simulink model "workingGT3nomasknwithcontrol"  (R2024a)
settings: Solver=ode15s  StartTime=0.0  StopTime=3600*48  RelTol=0.0001
model workspace (MAT data in the model file):
  TempGrad = 15
  Ti = 5
  roomarea1 = 20
libraries: fl_lib x2433, nesl_utility x241, SimscapeFluids_lib x137
(part 41 of 41)

== system workingGT3nomasknwithcontrol/OG2/Raum11/Heater/Controller fbh ==
  Temp : Inport
  Constant2 : Constant  Value=-1
  Product2 : Product
  Relay1 : Relay  OnSwitchValue=-19  OffSwitchValue=-21  OnOutputValue=.098  OffOutputValue=0.00001
  Simulink-PS Converter1 : nesl_utility/Simulink-PS Converter  PhysicalDomain=network_engine_domain  SubClassName=ps_input  LeftPortType=input  RightPortType=output  PseudoPeriodic=off  Frequencies=[]  NoiseDistribution=none  NoiseParameters=[]  Unit=1  AffineConversion=off  FilteringAndDerivatives=provide  SimscapeFilterOrder=1  InputFilterTimeConstant=0.001  UdotUserProvided=0
  output : PMIOPort  Side=Right
  wires:
  Constant2/1 -> Product2/2
  Temp/1 -> Product2/1
  Product2/1 -> Relay1/1
  Relay1/1 -> Simulink-PS Converter1/1
  connections:
  Simulink-PS Converter1/RConn1 -- output/RConn1

== system workingGT3nomasknwithcontrol/OG2/Raum12/Heater/Controller 11 ==
  In1 : Inport
  Constant2 : Constant  Value=-1
  Product2 : Product
  Relay1 : Relay  OnSwitchValue=-19  OffSwitchValue=-21  OnOutputValue=.095  OffOutputValue=0.00001
  Simulink-PS Converter1 : nesl_utility/Simulink-PS Converter  PhysicalDomain=network_engine_domain  SubClassName=ps_input  LeftPortType=input  RightPortType=output  PseudoPeriodic=off  Frequencies=[]  NoiseDistribution=none  NoiseParameters=[]  Unit=1  AffineConversion=off  FilteringAndDerivatives=provide  SimscapeFilterOrder=1  InputFilterTimeConstant=0.001  UdotUserProvided=0
  output : PMIOPort  Side=Right
  wires:
  Constant2/1 -> Product2/2
  In1/1 -> Product2/1
  Product2/1 -> Relay1/1
  Relay1/1 -> Simulink-PS Converter1/1
  connections:
  Simulink-PS Converter1/RConn1 -- output/RConn1

== system workingGT3nomasknwithcontrol/OG2/Raum12/Heater/Controller 22 ==
  Temp : Inport
  Constant2 : Constant  Value=-1
  Product2 : Product
  Relay1 : Relay  OnSwitchValue=-19  OffSwitchValue=-21  OnOutputValue=.098  OffOutputValue=0.00001
  Simulink-PS Converter1 : nesl_utility/Simulink-PS Converter  PhysicalDomain=network_engine_domain  SubClassName=ps_input  LeftPortType=input  RightPortType=output  PseudoPeriodic=off  Frequencies=[]  NoiseDistribution=none  NoiseParameters=[]  Unit=1  AffineConversion=off  FilteringAndDerivatives=provide  SimscapeFilterOrder=1  InputFilterTimeConstant=0.001  UdotUserProvided=0
  output : PMIOPort  Side=Right
  wires:
  Relay1/1 -> Simulink-PS Converter1/1
  Product2/1 -> Relay1/1
  Temp/1 -> Product2/1
  Constant2/1 -> Product2/2
  connections:
  Simulink-PS Converter1/RConn1 -- output/RConn1

== system workingGT3nomasknwithcontrol/OG2/Raum12/Heater/Controller 33 ==
  Temp : Inport
  Constant2 : Constant  Value=-1
  Product2 : Product
  Relay1 : Relay  OnSwitchValue=-19  OffSwitchValue=-21  OnOutputValue=.098  OffOutputValue=0.00001
  Simulink-PS Converter1 : nesl_utility/Simulink-PS Converter  PhysicalDomain=network_engine_domain  SubClassName=ps_input  LeftPortType=input  RightPortType=output  PseudoPeriodic=off  Frequencies=[]  NoiseDistribution=none  NoiseParameters=[]  Unit=1  AffineConversion=off  FilteringAndDerivatives=provide  SimscapeFilterOrder=1  InputFilterTimeConstant=0.001  UdotUserProvided=0
  output : PMIOPort  Side=Right
  wires:
  Constant2/1 -> Product2/2
  Temp/1 -> Product2/1
  Product2/1 -> Relay1/1
  Relay1/1 -> Simulink-PS Converter1/1
  connections:
  Simulink-PS Converter1/RConn1 -- output/RConn1

== system workingGT3nomasknwithcontrol/OG2/Raum12/Heater/Controller fbh ==
  Temp : Inport
  Constant2 : Constant  Value=-1
  Product2 : Product
  Relay1 : Relay  OnSwitchValue=-19  OffSwitchValue=-21  OnOutputValue=.098  OffOutputValue=0.00001
  Simulink-PS Converter1 : nesl_utility/Simulink-PS Converter  PhysicalDomain=network_engine_domain  SubClassName=ps_input  LeftPortType=input  RightPortType=output  PseudoPeriodic=off  Frequencies=[]  NoiseDistribution=none  NoiseParameters=[]  Unit=1  AffineConversion=off  FilteringAndDerivatives=provide  SimscapeFilterOrder=1  InputFilterTimeConstant=0.001  UdotUserProvided=0
  output : PMIOPort  Side=Right
  wires:
  Relay1/1 -> Simulink-PS Converter1/1
  Product2/1 -> Relay1/1
  Temp/1 -> Product2/1
  Constant2/1 -> Product2/2
  connections:
  Simulink-PS Converter1/RConn1 -- output/RConn1

== system workingGT3nomasknwithcontrol/OG2/Raum2/Heater/Controller 11 ==
  In1 : Inport
  Constant2 : Constant  Value=-1
  Product2 : Product
  Relay1 : Relay  OnSwitchValue=-14  OffSwitchValue=-16  OnOutputValue=.095  OffOutputValue=0.00001
  Simulink-PS Converter1 : nesl_utility/Simulink-PS Converter  PhysicalDomain=network_engine_domain  SubClassName=ps_input  LeftPortType=input  RightPortType=output  PseudoPeriodic=off  Frequencies=[]  NoiseDistribution=none  NoiseParameters=[]  Unit=1  AffineConversion=off  FilteringAndDerivatives=provide  SimscapeFilterOrder=1  InputFilterTimeConstant=0.001  UdotUserProvided=0
  output : PMIOPort  Side=Right
  wires:
  Constant2/1 -> Product2/2
  In1/1 -> Product2/1
  Product2/1 -> Relay1/1
  Relay1/1 -> Simulink-PS Converter1/1
  connections:
  Simulink-PS Converter1/RConn1 -- output/RConn1

== system workingGT3nomasknwithcontrol/OG2/Raum2/Heater/Controller 22 ==
  Temp : Inport
  Constant2 : Constant  Value=-1
  Product2 : Product
  Relay1 : Relay  OnSwitchValue=-19  OffSwitchValue=-21  OnOutputValue=.098  OffOutputValue=0.00001
  Simulink-PS Converter1 : nesl_utility/Simulink-PS Converter  PhysicalDomain=network_engine_domain  SubClassName=ps_input  LeftPortType=input  RightPortType=output  PseudoPeriodic=off  Frequencies=[]  NoiseDistribution=none  NoiseParameters=[]  Unit=1  AffineConversion=off  FilteringAndDerivatives=provide  SimscapeFilterOrder=1  InputFilterTimeConstant=0.001  UdotUserProvided=0
  output : PMIOPort  Side=Right
  wires:
  Relay1/1 -> Simulink-PS Converter1/1
  Product2/1 -> Relay1/1
  Temp/1 -> Product2/1
  Constant2/1 -> Product2/2
  connections:
  Simulink-PS Converter1/RConn1 -- output/RConn1

== system workingGT3nomasknwithcontrol/OG2/Raum2/Heater/Controller 33 ==
  Temp : Inport
  Constant2 : Constant  Value=-1
  Product2 : Product
  Relay1 : Relay  OnSwitchValue=-19  OffSwitchValue=-21  OnOutputValue=.098  OffOutputValue=0.00001
  Simulink-PS Converter1 : nesl_utility/Simulink-PS Converter  PhysicalDomain=network_engine_domain  SubClassName=ps_input  LeftPortType=input  RightPortType=output  PseudoPeriodic=off  Frequencies=[]  NoiseDistribution=none  NoiseParameters=[]  Unit=1  AffineConversion=off  FilteringAndDerivatives=provide  SimscapeFilterOrder=1  InputFilterTimeConstant=0.001  UdotUserProvided=0
  output : PMIOPort  Side=Right
  wires:
  Constant2/1 -> Product2/2
  Temp/1 -> Product2/1
  Product2/1 -> Relay1/1
  Relay1/1 -> Simulink-PS Converter1/1
  connections:
  Simulink-PS Converter1/RConn1 -- output/RConn1

== system workingGT3nomasknwithcontrol/OG2/Raum2/Heater/Controller fbh ==
  Temp : Inport
  Constant2 : Constant  Value=-1
  Product2 : Product
  Relay1 : Relay  OnSwitchValue=-19  OffSwitchValue=-21  OnOutputValue=.098  OffOutputValue=0.00001
  Simulink-PS Converter1 : nesl_utility/Simulink-PS Converter  PhysicalDomain=network_engine_domain  SubClassName=ps_input  LeftPortType=input  RightPortType=output  PseudoPeriodic=off  Frequencies=[]  NoiseDistribution=none  NoiseParameters=[]  Unit=1  AffineConversion=off  FilteringAndDerivatives=provide  SimscapeFilterOrder=1  InputFilterTimeConstant=0.001  UdotUserProvided=0
  output : PMIOPort  Side=Right
  wires:
  Relay1/1 -> Simulink-PS Converter1/1
  Product2/1 -> Relay1/1
  Temp/1 -> Product2/1
  Constant2/1 -> Product2/2
  connections:
  Simulink-PS Converter1/RConn1 -- output/RConn1

== system workingGT3nomasknwithcontrol/OG2/Raum3/Heater/Controller 11 ==
  In1 : Inport
  Constant2 : Constant  Value=-1
  Product2 : Product
  Relay1 : Relay  OnSwitchValue=-19  OffSwitchValue=-21  OnOutputValue=.095  OffOutputValue=0.00001
  Simulink-PS Converter1 : nesl_utility/Simulink-PS Converter  PhysicalDomain=network_engine_domain  SubClassName=ps_input  LeftPortType=input  RightPortType=output  PseudoPeriodic=off  Frequencies=[]  NoiseDistribution=none  NoiseParameters=[]  Unit=1  AffineConversion=off  FilteringAndDerivatives=provide  SimscapeFilterOrder=1  InputFilterTimeConstant=0.001  UdotUserProvided=0
  output : PMIOPort  Side=Right
  wires:
  Relay1/1 -> Simulink-PS Converter1/1
  Product2/1 -> Relay1/1
  In1/1 -> Product2/1
  Constant2/1 -> Product2/2
  connections:
  Simulink-PS Converter1/RConn1 -- output/RConn1

== system workingGT3nomasknwithcontrol/OG2/Raum3/Heater/Controller 22 ==
  Temp : Inport
  Constant2 : Constant  Value=-1
  Product2 : Product
  Relay1 : Relay  OnSwitchValue=-19  OffSwitchValue=-21  OnOutputValue=.098  OffOutputValue=0.00001
  Simulink-PS Converter1 : nesl_utility/Simulink-PS Converter  PhysicalDomain=network_engine_domain  SubClassName=ps_input  LeftPortType=input  RightPortType=output  PseudoPeriodic=off  Frequencies=[]  NoiseDistribution=none  NoiseParameters=[]  Unit=1  AffineConversion=off  FilteringAndDerivatives=provide  SimscapeFilterOrder=1  InputFilterTimeConstant=0.001  UdotUserProvided=0
  output : PMIOPort  Side=Right
  wires:
  Constant2/1 -> Product2/2
  Temp/1 -> Product2/1
  Product2/1 -> Relay1/1
  Relay1/1 -> Simulink-PS Converter1/1
  connections:
  Simulink-PS Converter1/RConn1 -- output/RConn1

== system workingGT3nomasknwithcontrol/OG2/Raum3/Heater/Controller 33 ==
  Temp : Inport
  Constant2 : Constant  Value=-1
  Product2 : Product
  Relay1 : Relay  OnSwitchValue=-19  OffSwitchValue=-21  OnOutputValue=.098  OffOutputValue=0.00001
  Simulink-PS Converter1 : nesl_utility/Simulink-PS Converter  PhysicalDomain=network_engine_domain  SubClassName=ps_input  LeftPortType=input  RightPortType=output  PseudoPeriodic=off  Frequencies=[]  NoiseDistribution=none  NoiseParameters=[]  Unit=1  AffineConversion=off  FilteringAndDerivatives=provide  SimscapeFilterOrder=1  InputFilterTimeConstant=0.001  UdotUserProvided=0
  output : PMIOPort  Side=Right
  wires:
  Relay1/1 -> Simulink-PS Converter1/1
  Product2/1 -> Relay1/1
  Temp/1 -> Product2/1
  Constant2/1 -> Product2/2
  connections:
  Simulink-PS Converter1/RConn1 -- output/RConn1

== system workingGT3nomasknwithcontrol/OG2/Raum3/Heater/Controller fbh ==
  Temp : Inport
  Constant2 : Constant  Value=-1
  Product2 : Product
  Relay1 : Relay  OnSwitchValue=-19  OffSwitchValue=-21  OnOutputValue=.098  OffOutputValue=0.00001
  Simulink-PS Converter1 : nesl_utility/Simulink-PS Converter  PhysicalDomain=network_engine_domain  SubClassName=ps_input  LeftPortType=input  RightPortType=output  PseudoPeriodic=off  Frequencies=[]  NoiseDistribution=none  NoiseParameters=[]  Unit=1  AffineConversion=off  FilteringAndDerivatives=provide  SimscapeFilterOrder=1  InputFilterTimeConstant=0.001  UdotUserProvided=0
  output : PMIOPort  Side=Right
  wires:
  Constant2/1 -> Product2/2
  Temp/1 -> Product2/1
  Product2/1 -> Relay1/1
  Relay1/1 -> Simulink-PS Converter1/1
  connections:
  Simulink-PS Converter1/RConn1 -- output/RConn1

== system workingGT3nomasknwithcontrol/OG2/Raum4/Heater/Controller 11 ==
  In1 : Inport
  Constant2 : Constant  Value=-1
  Product2 : Product
  Relay1 : Relay  OnSwitchValue=-23  OffSwitchValue=-25  OnOutputValue=.095  OffOutputValue=0.00001
  Simulink-PS Converter1 : nesl_utility/Simulink-PS Converter  PhysicalDomain=network_engine_domain  SubClassName=ps_input  LeftPortType=input  RightPortType=output  PseudoPeriodic=off  Frequencies=[]  NoiseDistribution=none  NoiseParameters=[]  Unit=1  AffineConversion=off  FilteringAndDerivatives=provide  SimscapeFilterOrder=1  InputFilterTimeConstant=0.001  UdotUserProvided=0
  output : PMIOPort  Side=Right
  wires:
  Relay1/1 -> Simulink-PS Converter1/1
  Product2/1 -> Relay1/1
  In1/1 -> Product2/1
  Constant2/1 -> Product2/2
  connections:
  Simulink-PS Converter1/RConn1 -- output/RConn1

== system workingGT3nomasknwithcontrol/OG2/Raum4/Heater/Controller 22 ==
  Temp : Inport
  Constant2 : Constant  Value=-1
  Product2 : Product
  Relay1 : Relay  OnSwitchValue=-19  OffSwitchValue=-21  OnOutputValue=.098  OffOutputValue=0.00001
  Simulink-PS Converter1 : nesl_utility/Simulink-PS Converter  PhysicalDomain=network_engine_domain  SubClassName=ps_input  LeftPortType=input  RightPortType=output  PseudoPeriodic=off  Frequencies=[]  NoiseDistribution=none  NoiseParameters=[]  Unit=1  AffineConversion=off  FilteringAndDerivatives=provide  SimscapeFilterOrder=1  InputFilterTimeConstant=0.001  UdotUserProvided=0
  output : PMIOPort  Side=Right
  wires:
  Constant2/1 -> Product2/2
  Temp/1 -> Product2/1
  Product2/1 -> Relay1/1
  Relay1/1 -> Simulink-PS Converter1/1
  connections:
  Simulink-PS Converter1/RConn1 -- output/RConn1

== system workingGT3nomasknwithcontrol/OG2/Raum4/Heater/Controller 33 ==
  Temp : Inport
  Constant2 : Constant  Value=-1
  Product2 : Product
  Relay1 : Relay  OnSwitchValue=-19  OffSwitchValue=-21  OnOutputValue=.098  OffOutputValue=0.00001
  Simulink-PS Converter1 : nesl_utility/Simulink-PS Converter  PhysicalDomain=network_engine_domain  SubClassName=ps_input  LeftPortType=input  RightPortType=output  PseudoPeriodic=off  Frequencies=[]  NoiseDistribution=none  NoiseParameters=[]  Unit=1  AffineConversion=off  FilteringAndDerivatives=provide  SimscapeFilterOrder=1  InputFilterTimeConstant=0.001  UdotUserProvided=0
  output : PMIOPort  Side=Right
  wires:
  Relay1/1 -> Simulink-PS Converter1/1
  Product2/1 -> Relay1/1
  Temp/1 -> Product2/1
  Constant2/1 -> Product2/2
  connections:
  Simulink-PS Converter1/RConn1 -- output/RConn1

== system workingGT3nomasknwithcontrol/OG2/Raum4/Heater/Controller fbh ==
  Temp : Inport
  Constant2 : Constant  Value=-1
  Product2 : Product
  Relay1 : Relay  OnSwitchValue=-19  OffSwitchValue=-21  OnOutputValue=.098  OffOutputValue=0.00001
  Simulink-PS Converter1 : nesl_utility/Simulink-PS Converter  PhysicalDomain=network_engine_domain  SubClassName=ps_input  LeftPortType=input  RightPortType=output  PseudoPeriodic=off  Frequencies=[]  NoiseDistribution=none  NoiseParameters=[]  Unit=1  AffineConversion=off  FilteringAndDerivatives=provide  SimscapeFilterOrder=1  InputFilterTimeConstant=0.001  UdotUserProvided=0
  output : PMIOPort  Side=Right
  wires:
  Constant2/1 -> Product2/2
  Temp/1 -> Product2/1
  Product2/1 -> Relay1/1
  Relay1/1 -> Simulink-PS Converter1/1
  connections:
  Simulink-PS Converter1/RConn1 -- output/RConn1

== system workingGT3nomasknwithcontrol/OG2/Raum5/Heater/Controller 11 ==
  In1 : Inport
  Constant2 : Constant  Value=-1
  Product2 : Product
  Relay1 : Relay  OnSwitchValue=-19  OffSwitchValue=-21  OnOutputValue=.095  OffOutputValue=0.00001
  Simulink-PS Converter1 : nesl_utility/Simulink-PS Converter  PhysicalDomain=network_engine_domain  SubClassName=ps_input  LeftPortType=input  RightPortType=output  PseudoPeriodic=off  Frequencies=[]  NoiseDistribution=none  NoiseParameters=[]  Unit=1  AffineConversion=off  FilteringAndDerivatives=provide  SimscapeFilterOrder=1  InputFilterTimeConstant=0.001  UdotUserProvided=0
  output : PMIOPort  Side=Right
  wires:
  Constant2/1 -> Product2/2
  In1/1 -> Product2/1
  Product2/1 -> Relay1/1
  Relay1/1 -> Simulink-PS Converter1/1
  connections:
  Simulink-PS Converter1/RConn1 -- output/RConn1

== system workingGT3nomasknwithcontrol/OG2/Raum5/Heater/Controller 22 ==
  Temp : Inport
  Constant2 : Constant  Value=-1
  Product2 : Product
  Relay1 : Relay  OnSwitchValue=-19  OffSwitchValue=-21  OnOutputValue=.098  OffOutputValue=0.00001
  Simulink-PS Converter1 : nesl_utility/Simulink-PS Converter  PhysicalDomain=network_engine_domain  SubClassName=ps_input  LeftPortType=input  RightPortType=output  PseudoPeriodic=off  Frequencies=[]  NoiseDistribution=none  NoiseParameters=[]  Unit=1  AffineConversion=off  FilteringAndDerivatives=provide  SimscapeFilterOrder=1  InputFilterTimeConstant=0.001  UdotUserProvided=0
  output : PMIOPort  Side=Right
  wires:
  Relay1/1 -> Simulink-PS Converter1/1
  Product2/1 -> Relay1/1
  Temp/1 -> Product2/1
  Constant2/1 -> Product2/2
  connections:
  Simulink-PS Converter1/RConn1 -- output/RConn1

== system workingGT3nomasknwithcontrol/OG2/Raum5/Heater/Controller 33 ==
  Temp : Inport
  Constant2 : Constant  Value=-1
  Product2 : Product
  Relay1 : Relay  OnSwitchValue=-19  OffSwitchValue=-21  OnOutputValue=.098  OffOutputValue=0.00001
  Simulink-PS Converter1 : nesl_utility/Simulink-PS Converter  PhysicalDomain=network_engine_domain  SubClassName=ps_input  LeftPortType=input  RightPortType=output  PseudoPeriodic=off  Frequencies=[]  NoiseDistribution=none  NoiseParameters=[]  Unit=1  AffineConversion=off  FilteringAndDerivatives=provide  SimscapeFilterOrder=1  InputFilterTimeConstant=0.001  UdotUserProvided=0
  output : PMIOPort  Side=Right
  wires:
  Constant2/1 -> Product2/2
  Temp/1 -> Product2/1
  Product2/1 -> Relay1/1
  Relay1/1 -> Simulink-PS Converter1/1
  connections:
  Simulink-PS Converter1/RConn1 -- output/RConn1

== system workingGT3nomasknwithcontrol/OG2/Raum5/Heater/Controller fbh ==
  Temp : Inport
  Constant2 : Constant  Value=-1
  Product2 : Product
  Relay1 : Relay  OnSwitchValue=-19  OffSwitchValue=-21  OnOutputValue=.098  OffOutputValue=0.00001
  Simulink-PS Converter1 : nesl_utility/Simulink-PS Converter  PhysicalDomain=network_engine_domain  SubClassName=ps_input  LeftPortType=input  RightPortType=output  PseudoPeriodic=off  Frequencies=[]  NoiseDistribution=none  NoiseParameters=[]  Unit=1  AffineConversion=off  FilteringAndDerivatives=provide  SimscapeFilterOrder=1  InputFilterTimeConstant=0.001  UdotUserProvided=0
  output : PMIOPort  Side=Right
  wires:
  Relay1/1 -> Simulink-PS Converter1/1
  Product2/1 -> Relay1/1
  Temp/1 -> Product2/1
  Constant2/1 -> Product2/2
  connections:
  Simulink-PS Converter1/RConn1 -- output/RConn1

== system workingGT3nomasknwithcontrol/OG2/Raum6/Heater/Controller 11 ==
  In1 : Inport
  Constant2 : Constant  Value=-1
  Product2 : Product
  Relay1 : Relay  OnSwitchValue=-19  OffSwitchValue=-21  OnOutputValue=.095  OffOutputValue=0.00001
  Simulink-PS Converter1 : nesl_utility/Simulink-PS Converter  PhysicalDomain=network_engine_domain  SubClassName=ps_input  LeftPortType=input  RightPortType=output  PseudoPeriodic=off  Frequencies=[]  NoiseDistribution=none  NoiseParameters=[]  Unit=1  AffineConversion=off  FilteringAndDerivatives=provide  SimscapeFilterOrder=1  InputFilterTimeConstant=0.001  UdotUserProvided=0
  output : PMIOPort  Side=Right
  wires:
  Relay1/1 -> Simulink-PS Converter1/1
  Product2/1 -> Relay1/1
  In1/1 -> Product2/1
  Constant2/1 -> Product2/2
  connections:
  Simulink-PS Converter1/RConn1 -- output/RConn1

== system workingGT3nomasknwithcontrol/OG2/Raum6/Heater/Controller 22 ==
  Temp : Inport
  Constant2 : Constant  Value=-1
  Product2 : Product
  Relay1 : Relay  OnSwitchValue=-19  OffSwitchValue=-21  OnOutputValue=.098  OffOutputValue=0.00001
  Simulink-PS Converter1 : nesl_utility/Simulink-PS Converter  PhysicalDomain=network_engine_domain  SubClassName=ps_input  LeftPortType=input  RightPortType=output  PseudoPeriodic=off  Frequencies=[]  NoiseDistribution=none  NoiseParameters=[]  Unit=1  AffineConversion=off  FilteringAndDerivatives=provide  SimscapeFilterOrder=1  InputFilterTimeConstant=0.001  UdotUserProvided=0
  output : PMIOPort  Side=Right
  wires:
  Constant2/1 -> Product2/2
  Temp/1 -> Product2/1
  Product2/1 -> Relay1/1
  Relay1/1 -> Simulink-PS Converter1/1
  connections:
  Simulink-PS Converter1/RConn1 -- output/RConn1

== system workingGT3nomasknwithcontrol/OG2/Raum6/Heater/Controller 33 ==
  Temp : Inport
  Constant2 : Constant  Value=-1
  Product2 : Product
  Relay1 : Relay  OnSwitchValue=-19  OffSwitchValue=-21  OnOutputValue=.098  OffOutputValue=0.00001
  Simulink-PS Converter1 : nesl_utility/Simulink-PS Converter  PhysicalDomain=network_engine_domain  SubClassName=ps_input  LeftPortType=input  RightPortType=output  PseudoPeriodic=off  Frequencies=[]  NoiseDistribution=none  NoiseParameters=[]  Unit=1  AffineConversion=off  FilteringAndDerivatives=provide  SimscapeFilterOrder=1  InputFilterTimeConstant=0.001  UdotUserProvided=0
  output : PMIOPort  Side=Right
  wires:
  Relay1/1 -> Simulink-PS Converter1/1
  Product2/1 -> Relay1/1
  Temp/1 -> Product2/1
  Constant2/1 -> Product2/2
  connections:
  Simulink-PS Converter1/RConn1 -- output/RConn1

== system workingGT3nomasknwithcontrol/OG2/Raum6/Heater/Controller fbh ==
  Temp : Inport
  Constant2 : Constant  Value=-1
  Product2 : Product
  Relay1 : Relay  OnSwitchValue=-19  OffSwitchValue=-21  OnOutputValue=.098  OffOutputValue=0.00001
  Simulink-PS Converter1 : nesl_utility/Simulink-PS Converter  PhysicalDomain=network_engine_domain  SubClassName=ps_input  LeftPortType=input  RightPortType=output  PseudoPeriodic=off  Frequencies=[]  NoiseDistribution=none  NoiseParameters=[]  Unit=1  AffineConversion=off  FilteringAndDerivatives=provide  SimscapeFilterOrder=1  InputFilterTimeConstant=0.001  UdotUserProvided=0
  output : PMIOPort  Side=Right
  wires:
  Constant2/1 -> Product2/2
  Temp/1 -> Product2/1
  Product2/1 -> Relay1/1
  Relay1/1 -> Simulink-PS Converter1/1
  connections:
  Simulink-PS Converter1/RConn1 -- output/RConn1

== system workingGT3nomasknwithcontrol/OG2/Raum7/Heater/Controller 11 ==
  In1 : Inport
  Constant2 : Constant  Value=-1
  Product2 : Product
  Relay1 : Relay  OnSwitchValue=-14  OffSwitchValue=-16  OnOutputValue=.095  OffOutputValue=0.00001
  Simulink-PS Converter1 : nesl_utility/Simulink-PS Converter  PhysicalDomain=network_engine_domain  SubClassName=ps_input  LeftPortType=input  RightPortType=output  PseudoPeriodic=off  Frequencies=[]  NoiseDistribution=none  NoiseParameters=[]  Unit=1  AffineConversion=off  FilteringAndDerivatives=provide  SimscapeFilterOrder=1  InputFilterTimeConstant=0.001  UdotUserProvided=0
  output : PMIOPort  Side=Right
  wires:
  Constant2/1 -> Product2/2
  In1/1 -> Product2/1
  Product2/1 -> Relay1/1
  Relay1/1 -> Simulink-PS Converter1/1
  connections:
  Simulink-PS Converter1/RConn1 -- output/RConn1

== system workingGT3nomasknwithcontrol/OG2/Raum7/Heater/Controller 22 ==
  Temp : Inport
  Constant2 : Constant  Value=-1
  Product2 : Product
  Relay1 : Relay  OnSwitchValue=-19  OffSwitchValue=-21  OnOutputValue=.098  OffOutputValue=0.00001
  Simulink-PS Converter1 : nesl_utility/Simulink-PS Converter  PhysicalDomain=network_engine_domain  SubClassName=ps_input  LeftPortType=input  RightPortType=output  PseudoPeriodic=off  Frequencies=[]  NoiseDistribution=none  NoiseParameters=[]  Unit=1  AffineConversion=off  FilteringAndDerivatives=provide  SimscapeFilterOrder=1  InputFilterTimeConstant=0.001  UdotUserProvided=0
  output : PMIOPort  Side=Right
  wires:
  Relay1/1 -> Simulink-PS Converter1/1
  Product2/1 -> Relay1/1
  Temp/1 -> Product2/1
  Constant2/1 -> Product2/2
  connections:
  Simulink-PS Converter1/RConn1 -- output/RConn1

== system workingGT3nomasknwithcontrol/OG2/Raum7/Heater/Controller 33 ==
  Temp : Inport
  Constant2 : Constant  Value=-1
  Product2 : Product
  Relay1 : Relay  OnSwitchValue=-19  OffSwitchValue=-21  OnOutputValue=.098  OffOutputValue=0.00001
  Simulink-PS Converter1 : nesl_utility/Simulink-PS Converter  PhysicalDomain=network_engine_domain  SubClassName=ps_input  LeftPortType=input  RightPortType=output  PseudoPeriodic=off  Frequencies=[]  NoiseDistribution=none  NoiseParameters=[]  Unit=1  AffineConversion=off  FilteringAndDerivatives=provide  SimscapeFilterOrder=1  InputFilterTimeConstant=0.001  UdotUserProvided=0
  output : PMIOPort  Side=Right
  wires:
  Constant2/1 -> Product2/2
  Temp/1 -> Product2/1
  Product2/1 -> Relay1/1
  Relay1/1 -> Simulink-PS Converter1/1
  connections:
  Simulink-PS Converter1/RConn1 -- output/RConn1

== system workingGT3nomasknwithcontrol/OG2/Raum7/Heater/Controller fbh ==
  Temp : Inport
  Constant2 : Constant  Value=-1
  Product2 : Product
  Relay1 : Relay  OnSwitchValue=-19  OffSwitchValue=-21  OnOutputValue=.098  OffOutputValue=0.00001
  Simulink-PS Converter1 : nesl_utility/Simulink-PS Converter  PhysicalDomain=network_engine_domain  SubClassName=ps_input  LeftPortType=input  RightPortType=output  PseudoPeriodic=off  Frequencies=[]  NoiseDistribution=none  NoiseParameters=[]  Unit=1  AffineConversion=off  FilteringAndDerivatives=provide  SimscapeFilterOrder=1  InputFilterTimeConstant=0.001  UdotUserProvided=0
  output : PMIOPort  Side=Right
  wires:
  Relay1/1 -> Simulink-PS Converter1/1
  Product2/1 -> Relay1/1
  Temp/1 -> Product2/1
  Constant2/1 -> Product2/2
  connections:
  Simulink-PS Converter1/RConn1 -- output/RConn1

== system workingGT3nomasknwithcontrol/OG2/Raum8/Heater/Controller 11 ==
  In1 : Inport
  Constant2 : Constant  Value=-1
  Product2 : Product
  Relay1 : Relay  OnSwitchValue=-23  OffSwitchValue=-25  OnOutputValue=.095  OffOutputValue=0.00001
  Simulink-PS Converter1 : nesl_utility/Simulink-PS Converter  PhysicalDomain=network_engine_domain  SubClassName=ps_input  LeftPortType=input  RightPortType=output  PseudoPeriodic=off  Frequencies=[]  NoiseDistribution=none  NoiseParameters=[]  Unit=1  AffineConversion=off  FilteringAndDerivatives=provide  SimscapeFilterOrder=1  InputFilterTimeConstant=0.001  UdotUserProvided=0
  output : PMIOPort  Side=Right
  wires:
  Constant2/1 -> Product2/2
  In1/1 -> Product2/1
  Product2/1 -> Relay1/1
  Relay1/1 -> Simulink-PS Converter1/1
  connections:
  Simulink-PS Converter1/RConn1 -- output/RConn1

== system workingGT3nomasknwithcontrol/OG2/Raum8/Heater/Controller 22 ==
  Temp : Inport
  Constant2 : Constant  Value=-1
  Product2 : Product
  Relay1 : Relay  OnSwitchValue=-19  OffSwitchValue=-21  OnOutputValue=.098  OffOutputValue=0.00001
  Simulink-PS Converter1 : nesl_utility/Simulink-PS Converter  PhysicalDomain=network_engine_domain  SubClassName=ps_input  LeftPortType=input  RightPortType=output  PseudoPeriodic=off  Frequencies=[]  NoiseDistribution=none  NoiseParameters=[]  Unit=1  AffineConversion=off  FilteringAndDerivatives=provide  SimscapeFilterOrder=1  InputFilterTimeConstant=0.001  UdotUserProvided=0
  output : PMIOPort  Side=Right
  wires:
  Relay1/1 -> Simulink-PS Converter1/1
  Product2/1 -> Relay1/1
  Temp/1 -> Product2/1
  Constant2/1 -> Product2/2
  connections:
  Simulink-PS Converter1/RConn1 -- output/RConn1

== system workingGT3nomasknwithcontrol/OG2/Raum8/Heater/Controller 33 ==
  Temp : Inport
  Constant2 : Constant  Value=-1
  Product2 : Product
  Relay1 : Relay  OnSwitchValue=-19  OffSwitchValue=-21  OnOutputValue=.098  OffOutputValue=0.00001
  Simulink-PS Converter1 : nesl_utility/Simulink-PS Converter  PhysicalDomain=network_engine_domain  SubClassName=ps_input  LeftPortType=input  RightPortType=output  PseudoPeriodic=off  Frequencies=[]  NoiseDistribution=none  NoiseParameters=[]  Unit=1  AffineConversion=off  FilteringAndDerivatives=provide  SimscapeFilterOrder=1  InputFilterTimeConstant=0.001  UdotUserProvided=0
  output : PMIOPort  Side=Right
  wires:
  Constant2/1 -> Product2/2
  Temp/1 -> Product2/1
  Product2/1 -> Relay1/1
  Relay1/1 -> Simulink-PS Converter1/1
  connections:
  Simulink-PS Converter1/RConn1 -- output/RConn1

== system workingGT3nomasknwithcontrol/OG2/Raum8/Heater/Controller fbh ==
  Temp : Inport
  Constant2 : Constant  Value=-1
  Product2 : Product
  Relay1 : Relay  OnSwitchValue=-19  OffSwitchValue=-21  OnOutputValue=.098  OffOutputValue=0.00001
  Simulink-PS Converter1 : nesl_utility/Simulink-PS Converter  PhysicalDomain=network_engine_domain  SubClassName=ps_input  LeftPortType=input  RightPortType=output  PseudoPeriodic=off  Frequencies=[]  NoiseDistribution=none  NoiseParameters=[]  Unit=1  AffineConversion=off  FilteringAndDerivatives=provide  SimscapeFilterOrder=1  InputFilterTimeConstant=0.001  UdotUserProvided=0
  output : PMIOPort  Side=Right
  wires:
  Relay1/1 -> Simulink-PS Converter1/1
  Product2/1 -> Relay1/1
  Temp/1 -> Product2/1
  Constant2/1 -> Product2/2
  connections:
  Simulink-PS Converter1/RConn1 -- output/RConn1

== system workingGT3nomasknwithcontrol/OG2/Raum9/Heater/Controller 11 ==
  In1 : Inport
  Constant2 : Constant  Value=-1
  Product2 : Product
  Relay1 : Relay  OnSwitchValue=-19  OffSwitchValue=-21  OnOutputValue=.095  OffOutputValue=0.00001
  Simulink-PS Converter1 : nesl_utility/Simulink-PS Converter  PhysicalDomain=network_engine_domain  SubClassName=ps_input  LeftPortType=input  RightPortType=output  PseudoPeriodic=off  Frequencies=[]  NoiseDistribution=none  NoiseParameters=[]  Unit=1  AffineConversion=off  FilteringAndDerivatives=provide  SimscapeFilterOrder=1  InputFilterTimeConstant=0.001  UdotUserProvided=0
  output : PMIOPort  Side=Right
  wires:
  Relay1/1 -> Simulink-PS Converter1/1
  Product2/1 -> Relay1/1
  In1/1 -> Product2/1
  Constant2/1 -> Product2/2
  connections:
  Simulink-PS Converter1/RConn1 -- output/RConn1

== system workingGT3nomasknwithcontrol/OG2/Raum9/Heater/Controller 22 ==
  Temp : Inport
  Constant2 : Constant  Value=-1
  Product2 : Product
  Relay1 : Relay  OnSwitchValue=-19  OffSwitchValue=-21  OnOutputValue=.098  OffOutputValue=0.00001
  Simulink-PS Converter1 : nesl_utility/Simulink-PS Converter  PhysicalDomain=network_engine_domain  SubClassName=ps_input  LeftPortType=input  RightPortType=output  PseudoPeriodic=off  Frequencies=[]  NoiseDistribution=none  NoiseParameters=[]  Unit=1  AffineConversion=off  FilteringAndDerivatives=provide  SimscapeFilterOrder=1  InputFilterTimeConstant=0.001  UdotUserProvided=0
  output : PMIOPort  Side=Right
  wires:
  Constant2/1 -> Product2/2
  Temp/1 -> Product2/1
  Product2/1 -> Relay1/1
  Relay1/1 -> Simulink-PS Converter1/1
  connections:
  Simulink-PS Converter1/RConn1 -- output/RConn1

== system workingGT3nomasknwithcontrol/OG2/Raum9/Heater/Controller 33 ==
  Temp : Inport
  Constant2 : Constant  Value=-1
  Product2 : Product
  Relay1 : Relay  OnSwitchValue=-19  OffSwitchValue=-21  OnOutputValue=.098  OffOutputValue=0.00001
  Simulink-PS Converter1 : nesl_utility/Simulink-PS Converter  PhysicalDomain=network_engine_domain  SubClassName=ps_input  LeftPortType=input  RightPortType=output  PseudoPeriodic=off  Frequencies=[]  NoiseDistribution=none  NoiseParameters=[]  Unit=1  AffineConversion=off  FilteringAndDerivatives=provide  SimscapeFilterOrder=1  InputFilterTimeConstant=0.001  UdotUserProvided=0
  output : PMIOPort  Side=Right
  wires:
  Relay1/1 -> Simulink-PS Converter1/1
  Product2/1 -> Relay1/1
  Temp/1 -> Product2/1
  Constant2/1 -> Product2/2
  connections:
  Simulink-PS Converter1/RConn1 -- output/RConn1

== system workingGT3nomasknwithcontrol/OG2/Raum9/Heater/Controller fbh ==
  Temp : Inport
  Constant2 : Constant  Value=-1
  Product2 : Product
  Relay1 : Relay  OnSwitchValue=-19  OffSwitchValue=-21  OnOutputValue=.098  OffOutputValue=0.00001
  Simulink-PS Converter1 : nesl_utility/Simulink-PS Converter  PhysicalDomain=network_engine_domain  SubClassName=ps_input  LeftPortType=input  RightPortType=output  PseudoPeriodic=off  Frequencies=[]  NoiseDistribution=none  NoiseParameters=[]  Unit=1  AffineConversion=off  FilteringAndDerivatives=provide  SimscapeFilterOrder=1  InputFilterTimeConstant=0.001  UdotUserProvided=0
  output : PMIOPort  Side=Right
  wires:
  Constant2/1 -> Product2/2
  Temp/1 -> Product2/1
  Product2/1 -> Relay1/1
  Relay1/1 -> Simulink-PS Converter1/1
  connections:
  Simulink-PS Converter1/RConn1 -- output/RConn1
